simulink model "L68"  (R2012b)
settings: Solver=ode45  StartTime=0.0  StopTime=30.0  RelTol=1e-3
values from neighbouring files (symbols this model uses):
  A = [0 1 0; 0 0 1; -22 -27 -33]    [t6.m]
  B = [0;0;14]    [t6.m]
  C = [1 0 0]    [t6.m]
  D = 0    [t6.m]
undefined symbols (not defined in the file or in its folder): A2, B2, C2, D2
settings Model: Creator=12105774  LastModifiedBy=13105129
settings DebuggingCC: FrameProcessingCompatibilityMsg=error
settings CodeAppCC: CustomSymbolStrType=$N$R$M_T
settings GRTTargetCC: CodeReplacementLibrary=C89/C90 (ANSI)

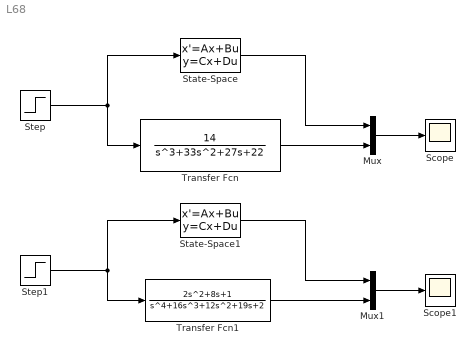
== system L68 ==
  Mux : Mux  Inputs=2
  Mux1 : Mux  Inputs=2
  Scope : Scope
      settings: ShowLegends=on  YMin=-10  YMax=10
  Scope1 : Scope
      settings: ShowLegends=on  YMin=-10  YMax=10
  State-Space : StateSpace  A=A  B=B  C=C  D=D
  State-Space1 : StateSpace  A=A2  B=B2  C=C2  D=D2
  Step : Step  SampleTime=0
  Step1 : Step  SampleTime=0
  Transfer Fcn : TransferFcn  Numerator=[14]  Denominator=[1 33 27 22]
  Transfer Fcn1 : TransferFcn  Numerator=[2 8 1]  Denominator=[1 16 12 19 2]
  wires:
  Transfer Fcn/1 -> Mux/2
  State-Space/1 -> Mux/1
  Step/1 -> Transfer Fcn/1, State-Space/1
  Mux/1 -> Scope/1
  Transfer Fcn1/1 -> Mux1/2
  State-Space1/1 -> Mux1/1
  Step1/1 -> Transfer Fcn1/1, State-Space1/1
  Mux1/1 -> Scope1/1
